simulink model "Pole_Placement"  (R2022b)
settings: Solver=VariableStepAuto  StartTime=0.0  StopTime=10.0  RelTol=1e-3
values from neighbouring files (symbols this model uses):
  A = [0 0 1 0 ... (first row only)    [Unstable_Position.m]
  B = kt * B / Rm    [Unstable_Position.m]
  C = eye(2,4)    [Unstable_Position.m]
  K = place(A,B,P)    [Unstable_Position.m]
settings Model: Creator=Luca Faccioli  LastModifiedBy=Luca Faccioli

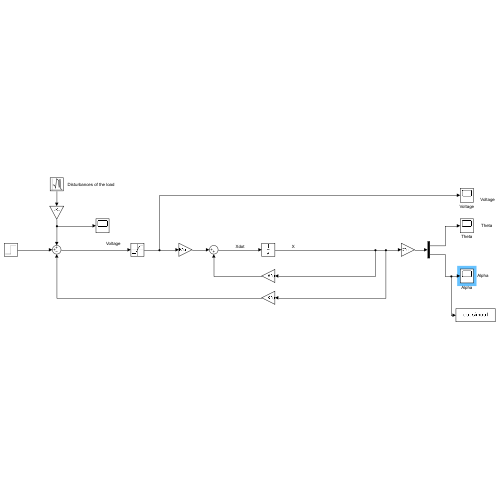
[thumbnail: Simulink's stored preview of the top-level diagram]
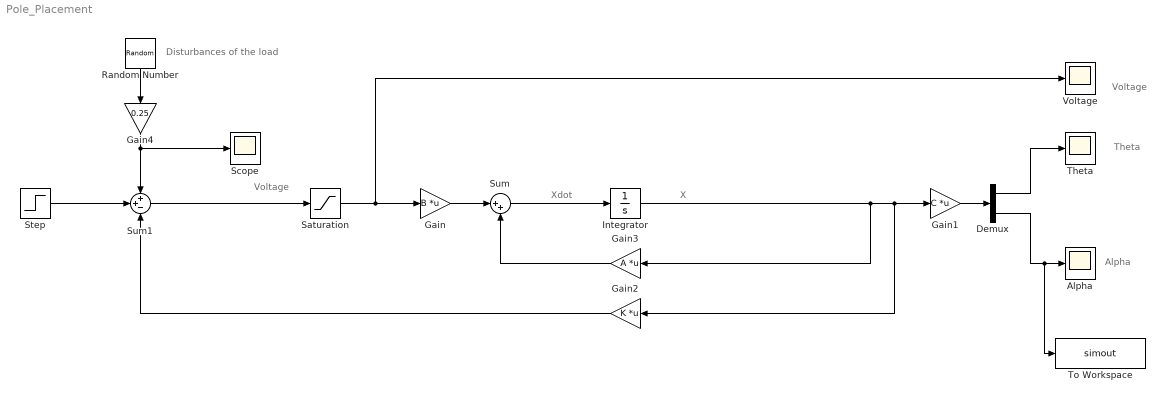
== system Pole_Placement ==
  note: Disturbances of the load
  note: Voltage
  note: Theta
  note: Alpha
  note: Voltage
  note: Xdot
  note: X
  Alpha : Scope
  Demux : Demux  Outputs=2
  Gain : Gain  Gain=B  Multiplication=Matrix(K*u)
  Gain1 : Gain  Gain=C  Multiplication=Matrix(K*u)
  Gain2 : Gain  Gain=K  Multiplication=Matrix(K*u)
  Gain3 : Gain  Gain=A  Multiplication=Matrix(K*u)
  Gain4 : Gain  Gain=0.25
  Integrator : Integrator  InitialCondition=[0,10*pi/180,0,0]
  Random Number : RandomNumber  SampleTime=0.05
  Saturation : Saturate  UpperLimit=10  LowerLimit=-10
  Scope : Scope
  Step : Step  Time=0  After=0  SampleTime=0.05
  Sum : Sum  Inputs=|++
  Sum1 : Sum  Inputs=++-
  Theta : Scope
  To Workspace : ToWorkspace  VariableName=simout  SampleTime=-1
  Voltage : Scope
  wires:
  Gain/1 -> Sum/1
  Sum/1 -> Integrator/1
  Gain1/1 -> Demux/1
  Demux/1 -> Theta/1
  Demux/2 -> To Workspace/1, Alpha/1
  Gain2/1 -> Sum1/3
  Sum1/1 -> Saturation/1
  Gain3/1 -> Sum/2
  Integrator/1 -> Gain3/1, Gain2/1, Gain1/1
  Saturation/1 -> Voltage/1, Gain/1
  Step/1 -> Sum1/2
  Random Number/1 -> Gain4/1
  Gain4/1 -> Sum1/1, Scope/1
